simulink model "es2_sim"  (R2023b)
settings: Solver=VariableStepAuto  StartTime=0.0  StopTime=10.0  RelTol=1e-3
values from neighbouring files (symbols this model uses):
  ueq = 0    [es2.m]
settings Model: Creator=stefa  LastModifiedBy=stefa

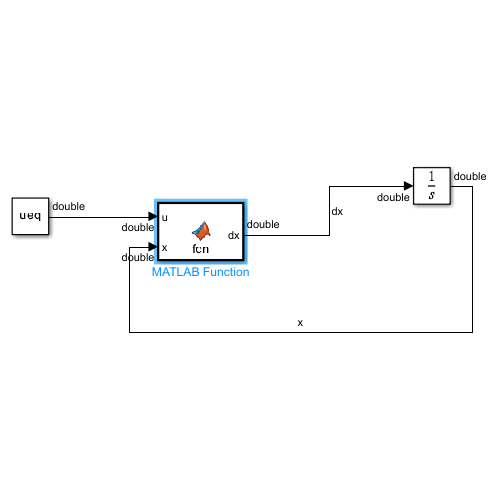
[thumbnail: Simulink's stored preview of the top-level diagram]
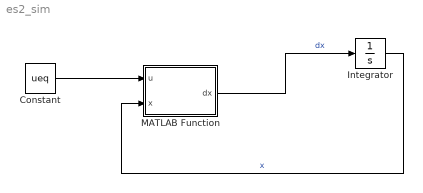
== system es2_sim ==
  Constant : Constant  Value=ueq
  Integrator : Integrator
  MATLAB Function : MATLAB Function  TreatAsAtomicUnit=on
  wires:
  MATLAB Function/1(dx) -> Integrator/1  "dx"
  Integrator/1 -> MATLAB Function/2(x)  "x"
  Constant/1 -> MATLAB Function/1(u)

== matlab function es2_sim/MATLAB Function ==
  data: u input; dx output; x input
function dx = fcn(u,x)
x1=x(1);
x2=x(2);
dx = [-x1+6*cos(x2);(x2^2+x2)*x1-x1*u+6*cos(x1)*u];
